simulink model "part2"  (R2025b)
settings: Solver=FixedStepAuto  StartTime=0.0  StopTime=500  FixedStep=0.1  RelTol=1e-3
values from neighbouring files (symbols this model uses):
  Aw = [zeros(3) eye(3); -diag_natwavefreq^2 -2*diag_reldampratios*diag_natwavefreq]    [NPO_init.m]    (also in kalman_init.m; passive_observer_init.m)
  Cw = [zeros(3) eye(3)]    [NPO_init.m]    (also in kalman_init.m; passive_observer_init.m)
  D = [2.6486e5 0 0 ... (first row only)    [NPO_init.m]    (also in kalman_init.m; passive_observer_init.m)
  h = 0.1    [init.m]
  K1 = [ diag([k1 k2 k3]) ... (first row only)    [NPO_init.m]    (also in passive_observer_init.m)
  K2 = diag([k7 k8 k9])    [NPO_init.m]    (also in passive_observer_init.m)
  K3 = 0.1*K4    [NPO_init.m]    (also in passive_observer_init.m = diag(diag(M) * 1e-1))
  K4 = diag([ 1000 10000 1000])    [NPO_init.m]    (also in passive_observer_init.m = diag(diag(M)))
  K_d = 2*M*Z*OMEGA_n    [init_controller.m]
  K_i = 0.1*K_p*OMEGA_n    [init_controller.m]
  K_p = M*OMEGA_n^2    [init_controller.m]
  M_inv = vesselABC.Minv([1 2 6], [1 2 6])    [NPO_init.m]    (also in kalman_init.m; passive_observer_init.m)
  T = diag([10000, 10000, 100])    [NPO_init.m]    (also in passive_observer_init.m = diag([100, 100, 100]))
  thrusters =     [thrusters_sup.mat]
  vessel =     [supply.mat]
undefined symbols (not defined in the file or in its folder): Hoerner
libraries: marine_gnc x2, marine_hydro x2
settings Model: Creator=jonbjor  LastModifiedBy=User
settings SolverCC: AlgebraicLoopSolver=TrustRegion
settings DataIOCC: ReturnWorkspaceOutputs=off
settings DebuggingCC: UnconnectedInputMsg=warning  UnconnectedOutputMsg=warning  UnconnectedLineMsg=warning  ArithmeticOperatorsInVariantConditions=warning
settings ModelReferenceCC: EnableRefExpFcnMdlSchedulingChecks=on
settings SFSimCC: SimUseLocalCustomCode=off  CustomCodeUndefinedFunction=UseInterfaceOnly
settings RTWCC: RTWUseLocalCustomCode=off  GPUComputeCapability=3.5  DLArmComputeVersion=19.05

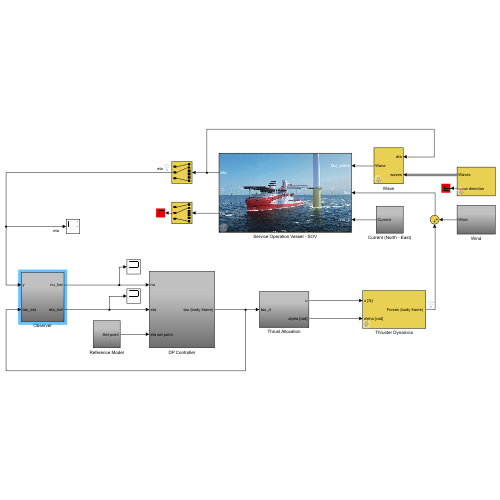
[thumbnail: Simulink's stored preview of the top-level diagram]
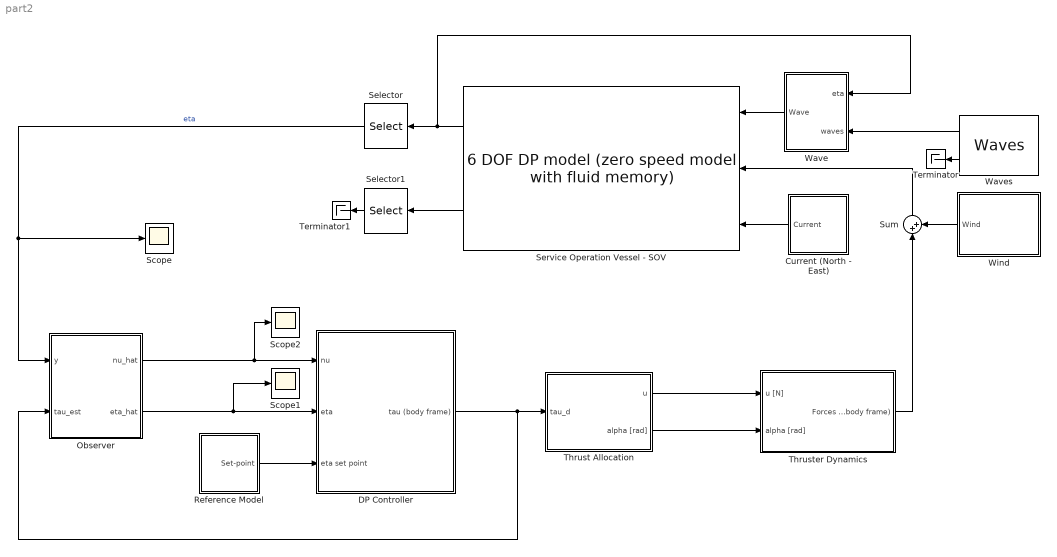
== system part2 ==
  Current (North - East) : Subsystem
  DP Controller : Subsystem
  Observer : Subsystem
  Reference Model : Subsystem
  Scope : Scope
      settings: ActiveDisplayYMinimum=-5.6386509566792773  ActiveDisplayYMaximum=19.827178567067236
  Scope1 : Scope
      settings: ActiveDisplayYMinimum=-7.2763512217109962  ActiveDisplayYMaximum=4.2414484621942279
  Scope2 : Scope
      settings: ActiveDisplayYMinimum=-5.4085848942959505  ActiveDisplayYMaximum=19.437811598484206  DataLoggingVariableName=ScopeData2
  Selector : Selector  InputPortWidth=6  IndexOptions=Index vector (dialog)  Indices=[1 2 6]  OutputSizes=1
  Selector1 : Selector  InputPortWidth=6  IndexOptions=Index vector (dialog)  Indices=[1 2 6]  OutputSizes=1
  Service Operation Vessel - SOV : marine_hydro/Hydro Library/6 DOF DP model  (zero speed model with fluid memory)  ABC=vesselABC  rho=1025  Axc=0.9*vessel.main.T*vessel.main.B  Ayc=0.9*vessel.main.T*vessel.main.Lpp  CX=1  CY_2D=Hoerner(vessel.main.B,vessel.main.T)  Bv=vessel.Bv  mask(6 DOF zero speed model){}
      link override "Integrator1 ": InitialCondition=nu0
      link override Integrator2: InitialCondition=eta0
      settings: SourceProductName=MSS Hydro
      mask Display:
      | image('SOV.jpg');
      | color('white'); port_label('output', 1, 'eta')
      | color('white'); port_label('output', 2, 'nu')
      | color('white'); port_label('input', 1, 'tau_wave')
      | color('white'); port_label('input', 2, 'tau')
      | color('white'); port_label('input', 3, 'nu_c')
  Sum : Sum  Inputs=|++
  Terminator : Terminator
  Terminator1 : Terminator
  Thrust Allocation : Subsystem
  Thruster Dynamics : Subsystem  mask{thrusterfault=off}
      mask prompts: thrusterfault "Fault on thruster #2 and #4?"
  Wave : Subsystem  mask{waveforces=on}
      mask prompts: waveforces "Waveforces enabled"
  Waves : marine_gnc/Environment/Waves/Waves  spectrum_type=ITTC  disp_flag=on  plot_spectrum=off  plot_realization=off  hs=2.5  omega_peak=2*pi/9  psi_mean=0  gamma=-1  spread=2  depth=inf  nfreq=20  ndir=10  energylim=0.005  freq_cutoff=3  dir_cutoff=0  rand_seed=123  rand_freq=on  rand_dir=on  Zeta_a=0  Omega=0  Phase=0  Wavenum=0  Psi=0
      settings: SourceProductName=MSS GNC
  Wind : Subsystem
  wires:
  Service Operation Vessel - SOV/2 -> Selector1/1
  Reference Model/1(Set-point) -> DP Controller/3(eta set point)
  DP Controller/1(tau (body frame)) -> Thrust Allocation/1(tau_d), Observer/2(tau_est)
  Service Operation Vessel - SOV/1 -> Wave/1(eta), Selector/1
  Current (North - East)/1(Current) -> Service Operation Vessel - SOV/3
  Wave/1(Wave) -> Service Operation Vessel - SOV/1
  Waves/1 -> Wave/2(waves)
  Waves/2 -> Terminator/1
  Selector1/1 -> Terminator1/1
  Observer/2(eta_hat) -> Scope1/1, DP Controller/2(eta)
  Observer/1(nu_hat) -> Scope2/1, DP Controller/1(nu)
  Thrust Allocation/1(u) -> Thruster Dynamics/1(u [N])
  Wind/1(Wind) -> Sum/2
  Thruster Dynamics/1("Forces (body frame) ") -> Sum/1
  Sum/1 -> Service Operation Vessel - SOV/2
  Thrust Allocation/2(alpha [rad]) -> Thruster Dynamics/2(alpha [rad])
  Selector/1 -> Scope/1, Observer/1(y)  "eta"

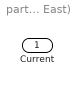
== system part2/Current (North - East) ==
  Current : Outport  VectorParamsAs1DForOutWhenUnconnected=off

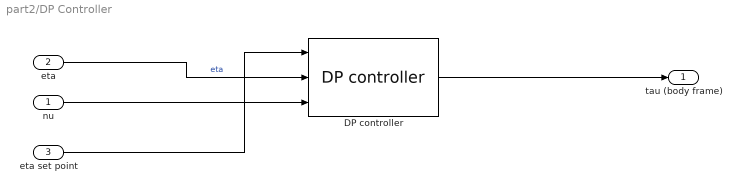
== system part2/DP Controller ==
  nu : Inport
  eta : Inport  Port=2
  eta set point : Inport  Port=3
  DP controller : marine_gnc/Control/Dynamic  Positioning /DP controller  Kp=K_p  Kd=K_d  Ki=K_i
      settings: SourceProductName=MSS GNC
  tau (body frame) : Outport  VectorParamsAs1DForOutWhenUnconnected=off
  wires:
  eta/1 -> DP controller/2  "eta"
  nu/1 -> DP controller/3
  eta set point/1 -> DP controller/1
  DP controller/1 -> tau (body frame)/1

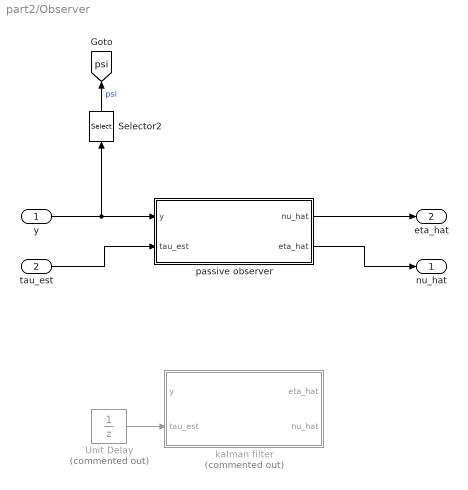
== system part2/Observer ==
  y : Inport
  tau_est : Inport  Port=2
  Selector2 : Selector  InputPortWidth=3  IndexOptions=Index vector (dialog)  Indices=[3]  OutputSizes=1
  Unit Delay : UnitDelay  Commented=on  SampleTime=h  HasFrameUpgradeWarning=on
  kalman filter : MATLAB Function  Commented=on  TreatAsAtomicUnit=on
  passive observer : Subsystem
  nu_hat : Outport  VectorParamsAs1DForOutWhenUnconnected=off
  eta_hat : Outport  Port=2  VectorParamsAs1DForOutWhenUnconnected=off
  tag scope: psi=global
  wires:
  Unit Delay/1 -> kalman filter/2(tau_est)
  Selector2/1 -> [psi]  "psi"
  y/1 -> Selector2/1, passive observer/1(y)
  passive observer/2(eta_hat) -> nu_hat/1
  passive observer/1(nu_hat) -> eta_hat/1
  tau_est/1 -> passive observer/2(tau_est)

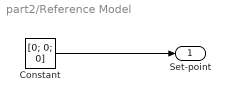
== system part2/Reference Model ==
  Constant : Constant  Value=[0; 0; 0]
  Set-point : Outport  VectorParamsAs1DForOutWhenUnconnected=off
  wires:
  Constant/1 -> Set-point/1

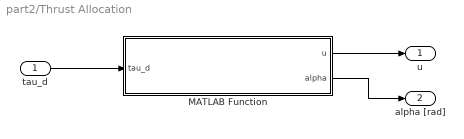
== system part2/Thrust Allocation ==
  tau_d : Inport
  MATLAB Function : MATLAB Function  TreatAsAtomicUnit=on
  u : Outport  VectorParamsAs1DForOutWhenUnconnected=off
  alpha [rad] : Outport  Port=2  VectorParamsAs1DForOutWhenUnconnected=off
  wires:
  tau_d/1 -> MATLAB Function/1(tau_d)
  MATLAB Function/1(u) -> u/1
  MATLAB Function/2(alpha) -> alpha [rad]/1

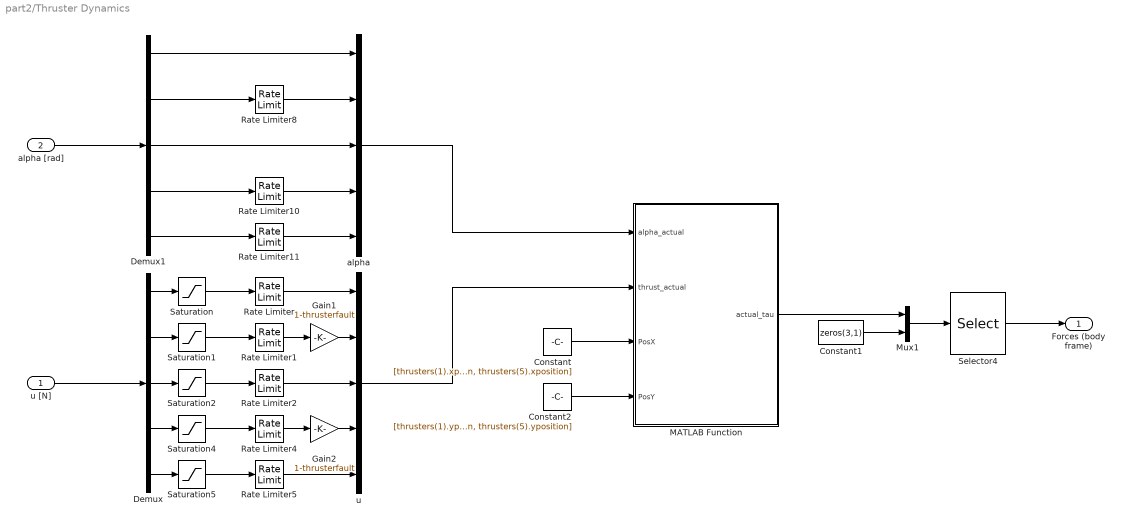
== system part2/Thruster Dynamics ==
  u [N] : Inport
  alpha [rad] : Inport  Port=2
  Constant : Constant  Value=[thrusters(1).xposition, thrusters(2).xposition, thrusters(3).xposition, thrusters(4).xposition, thrusters(5).xposition]
  Constant1 : Constant  Value=zeros(3,1)
  Constant2 : Constant  Value=[thrusters(1).yposition, thrusters(2).yposition, thrusters(3).yposition, thrusters(4).yposition, thrusters(5).yposition]
  Demux : Demux  Outputs=5
  Demux1 : Demux  Outputs=5
  Gain1 : Gain  Gain=1-thrusterfault
  Gain2 : Gain  Gain=1-thrusterfault
  MATLAB Function : MATLAB Function  TreatAsAtomicUnit=on
  Mux1 : Mux  Inputs=2
  Rate Limiter : RateLimiter  RisingSlewLimit=thrusters(1).rate  FallingSlewLimit=-thrusters(1).rate  SampleTimeMode=inherited
  Rate Limiter1 : RateLimiter  RisingSlewLimit=thrusters(2).rate  FallingSlewLimit=-thrusters(2).rate  SampleTimeMode=inherited
  Rate Limiter10 : RateLimiter  RisingSlewLimit=thrusters(4).rotationspeed  FallingSlewLimit=-thrusters(4).rotationspeed  SampleTimeMode=inherited
  Rate Limiter11 : RateLimiter  RisingSlewLimit=thrusters(5).rotationspeed  FallingSlewLimit=-thrusters(5).rotationspeed  SampleTimeMode=inherited
  Rate Limiter2 : RateLimiter  RisingSlewLimit=thrusters(3).rate  FallingSlewLimit=-thrusters(3).rate  SampleTimeMode=inherited
  Rate Limiter4 : RateLimiter  RisingSlewLimit=thrusters(4).rate  FallingSlewLimit=-thrusters(4).rate  SampleTimeMode=inherited
  Rate Limiter5 : RateLimiter  RisingSlewLimit=thrusters(5).rate  FallingSlewLimit=-thrusters(5).rate  SampleTimeMode=inherited
  Rate Limiter8 : RateLimiter  RisingSlewLimit=thrusters(2).rotationspeed  FallingSlewLimit=-thrusters(2).rotationspeed  SampleTimeMode=inherited
  Saturation : Saturate  UpperLimit=thrusters(1).thrust  LowerLimit=-thrusters(1).thrust
  Saturation1 : Saturate  UpperLimit=thrusters(2).thrust  LowerLimit=-thrusters(2).thrust
  Saturation2 : Saturate  UpperLimit=thrusters(3).thrust  LowerLimit=-thrusters(3).thrust
  Saturation4 : Saturate  UpperLimit=thrusters(4).thrust  LowerLimit=-thrusters(4).thrust
  Saturation5 : Saturate  UpperLimit=thrusters(5).thrust  LowerLimit=-thrusters(5).thrust
  Selector4 : Selector  InputPortWidth=6  IndexOptions=Index vector (dialog)  Indices=[1 2 4 5 6 3]  OutputSizes=1
  alpha : Mux  Inputs=5
  u : Mux  Inputs=5
  "Forces (body frame) " : Outport  VectorParamsAs1DForOutWhenUnconnected=off
  wires:
  Rate Limiter2/1 -> u/3
  Saturation/1 -> Rate Limiter/1
  Mux1/1 -> Selector4/1
  Constant1/1 -> Mux1/2
  Saturation4/1 -> Rate Limiter4/1
  Demux/2 -> Saturation1/1
  Saturation1/1 -> Rate Limiter1/1
  Demux/1 -> Saturation/1
  Demux/3 -> Saturation2/1
  Saturation2/1 -> Rate Limiter2/1
  Selector4/1 -> "Forces (body frame) "/1
  Gain1/1 -> u/2
  Rate Limiter1/1 -> Gain1/1
  Rate Limiter/1 -> u/1
  Rate Limiter4/1 -> Gain2/1
  Saturation5/1 -> Rate Limiter5/1
  u [N]/1 -> Demux/1
  alpha [rad]/1 -> Demux1/1
  Constant/1 -> MATLAB Function/3(PosX)
  Constant2/1 -> MATLAB Function/4(PosY)
  u/1 -> MATLAB Function/2(thrust_actual)
  alpha/1 -> MATLAB Function/1(alpha_actual)
  MATLAB Function/1(actual_tau) -> Mux1/1
  Rate Limiter10/1 -> alpha/4
  Demux1/4 -> Rate Limiter10/1
  Demux1/5 -> Rate Limiter11/1
  Rate Limiter11/1 -> alpha/5
  Demux1/1 -> alpha/1
  Gain2/1 -> u/4
  Demux/4 -> Saturation4/1
  Demux/5 -> Saturation5/1
  Rate Limiter5/1 -> u/5
  Demux1/2 -> Rate Limiter8/1
  Rate Limiter8/1 -> alpha/2
  Demux1/3 -> alpha/3

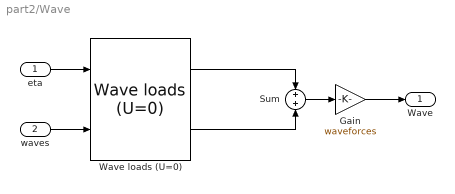
== system part2/Wave ==
  eta : Inport
  waves : Inport  Port=2
  Gain : Gain  Gain=waveforces
  Sum : Sum
  Wave loads (U=0) : marine_hydro/Hydro Library/Wave loads (U=0)  SystemSampleTime=-1  VariantActivationTime=update diagram  EmptyChoice=off  PassThrough=off  PassThroughVariantControl=(default)  EmptyChoiceVariantControl=(default)  AllowFlexibleInterface=on  Latency=0  AutoFrameSizeCalculation=off
  Wave : Outport  VectorParamsAs1DForOutWhenUnconnected=off
  wires:
  eta/1 -> Wave loads (U=0)/1
  waves/1 -> Wave loads (U=0)/2
  Sum/1 -> Gain/1
  Wave loads (U=0)/1 -> Sum/1
  Wave loads (U=0)/2 -> Sum/2
  Gain/1 -> Wave/1

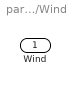
== system part2/Wind ==
  Wind : Outport  VectorParamsAs1DForOutWhenUnconnected=off

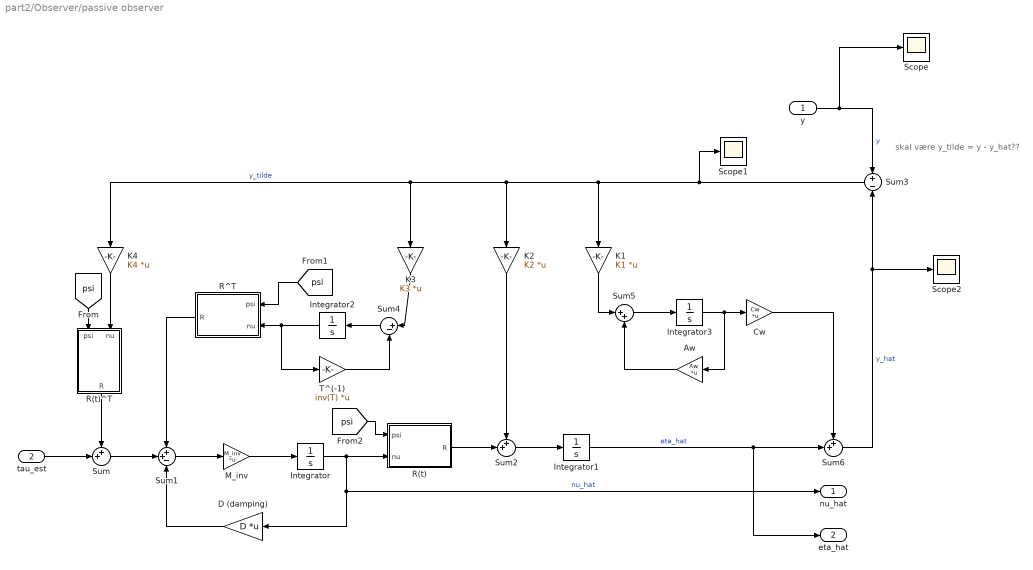
== system part2/Observer/passive observer ==
  note: skal være y_tilde = y - y_hat??
  y : Inport
  tau_est : Inport  Port=2
  Aw : Gain  Gain=Aw  Multiplication=Matrix(K*u)
  Cw : Gain  Gain=Cw  Multiplication=Matrix(K*u)
  D (damping) : Gain  Gain=D  Multiplication=Matrix(K*u)
  Integrator{,1..3} (4 alike) : Integrator
  K1 : Gain  Gain=K1  Multiplication=Matrix(K*u)
  K2 : Gain  Gain=K2  Multiplication=Matrix(K*u)
  K3 : Gain  Gain=K3  Multiplication=Matrix(K*u)
  K4 : Gain  Gain=K4  Multiplication=Matrix(K*u)
  M_inv : Gain  Gain=M_inv  Multiplication=Matrix(K*u)
  R(t) : MATLAB Function  TreatAsAtomicUnit=on
  R(t)^T : MATLAB Function  TreatAsAtomicUnit=on
  R^T : MATLAB Function  TreatAsAtomicUnit=on
  Scope : Scope
      settings: ActiveDisplayYMinimum=-5.6386509566792773  ActiveDisplayYMaximum=19.827178567067236  DataLoggingVariableName=ScopeData3
  Scope1 : Scope
      settings: ActiveDisplayYMinimum=-0.32989192595457506  ActiveDisplayYMaximum=0.716715390068409  DataLoggingVariableName=ScopeData4
  Scope2 : Scope
      settings: ActiveDisplayYMinimum=-5.4085848942959505  ActiveDisplayYMaximum=19.437811598484206  DataLoggingVariableName=ScopeData5
  Sum : Sum  Inputs=++|
  Sum1 : Sum  Inputs=++-
  Sum2 : Sum  Inputs=++|
  Sum3 : Sum  Inputs=+|-
  Sum4 : Sum  Inputs=|+-
  Sum5 : Sum  Inputs=|++
  Sum6 : Sum  Inputs=++|
  T^(-1) : Gain  Gain=inv(T)  Multiplication=Matrix(K*u)
  nu_hat : Outport  Unit=Inherit  PortDimensions=3
  eta_hat : Outport  Port=2  Unit=Inherit  PortDimensions=3
  wires:
  tau_est/1 -> Sum/2
  Sum/1 -> Sum1/2
  Sum1/1 -> M_inv/1
  M_inv/1 -> Integrator/1
  Integrator/1 -> R(t)/2(nu), D (damping)/1, nu_hat/1  "nu_hat"
  D (damping)/1 -> Sum1/3
  Sum2/1 -> Integrator1/1
  Integrator1/1 -> eta_hat/1, Sum6/2  "eta_hat"
  K2/1 -> Sum2/1
  y/1 -> Scope/1, Sum3/1  "y"
  K4/1 -> R(t)^T/2(nu)
  R(t)^T/1(R) -> Sum/1
  R(t)/1(R) -> Sum2/2
  Integrator2/1 -> T^(-1)/1, R^T/2(nu)
  Sum4/1 -> Integrator2/1
  T^(-1)/1 -> Sum4/2
  K3/1 -> Sum4/1
  R^T/1(R) -> Sum1/1
  Sum5/1 -> Integrator3/1
  Aw/1 -> Sum5/2
  K1/1 -> Sum5/1
  Integrator3/1 -> Aw/1, Cw/1
  Sum6/1 -> Scope2/1, Sum3/2  "y_hat"
  Sum3/1 -> Scope1/1, K1/1, K2/1, K3/1, K4/1  "y_tilde"
  Cw/1 -> Sum6/1
  [psi] -> R(t)^T/1(psi)
  [psi] -> R^T/1(psi)
  [psi] -> R(t)/1(psi)

== matlab function part2/Thrust Allocation/MATLAB Function ==
  data: tau_d input; u output; alpha output
function [u, alpha] = thrust_allocation_simplified(tau_d)
% INPUTS:  tau_d = [Fx; Fy; Mz] - Desired forces/moment (3x1)
% OUTPUTS: u = [u1; u2; u3; u4; u5] - Thrust magnitudes (5x1) [N]
%          alpha = [90; α2; 90; α4; α5] - Thruster angles (5x1) [deg]

%% Thruster Configuration
% Positions [m]
x = [39.3, 36.5, 34.3, -28.5, -28.5];  % x-coordinates
y = [0, 0, 0, 5, -5];                   % y-coordinates

%% Build B Matrix (3x8) - Force Decomposition
% Matrix structure: [T1, T2x, T2y, T3, T4x, T4y, T5x, T5y]
% Matrix structure: [T1, T2x, T2y, T3, T4x, T4y, T5x, T5y]
B = [
    0     1     0     0     1     0     1     0;  % Surge forces  
    1     0     1     1     0     1     0     1;  % Sway forces    
    x(1) -y(2)  x(2)  x(3) -y(4)  x(4) -y(5)  x(5)]; % Yaw moments

%% Solve using Pseudo-Inverse (Minimum-Norm Solution)
u_forces = pinv(B) * tau_d;

%% Extract Force Components
u1 = u_forces(1);      % T1 tunnel
u2x = u_forces(2);     % T2 surge component
u2y = u_forces(3);     % T2 sway component
u3 = u_forces(4);      % T3 tunnel
u4x = u_forces(5);     % T4 surge component
u4y = u_forces(6);     % T4 sway component
u5x = u_forces(7);     % T5 surge component
u5y = u_forces(8);     % T5 sway component

%% Convert to Thruster Commands
% Output vectors
u = zeros(5, 1);
alpha = zeros(5, 1);

% T1: Fixed tunnel at 90°
u(1) = u1;
alpha(1) = 90;

% T2: Variable azimuth
u(2) = sqrt(u2x^2 + u2y^2);
if u2x ~= 0 || u2y ~= 0
    alpha(2) = atan2d(u2y, u2x);
else
    alpha(2) = 0;
end

% T3: Fixed tunnel at 90°
u(3) = u3;
alpha(3) = 90;

% T4: Variable azimuth
u(4) = sqrt(u4x^2 + u4y^2);
if u4x ~= 0 || u4y ~= 0
    alpha(4) = atan2d(u4y, u4x);
else
    alpha(4) = 0;
end

% T5: Variable azimuth
u(5) = sqrt(u5x^2 + u5y^2);
if u5x ~= 0 || u5y ~= 0
    alpha(5) = atan2d(u5y, u5x);
else
    alpha(5) = 0;
end

== matlab function part2/Observer/kalman filter ==
  settings: updateMethod=DISCRETE  sampleTime=h
  data: y input; eta_hat output; tau_est input; nu_hat output
function [eta_hat, nu_hat] = kalman_filter(y, tau_est)

persistent x_prd P_prd
persistent isInitialized

if isempty(isInitialized)
    x_prd = zeros(15,1);
    P_prd = zeros(15); %eye(15)*1e-3;
    isInitialized = true;
end

h = 0.1;

M = [7.0184e6 0 0;
     0 8.5464e6 -4.4678e7;
     0 -4.5028e5 4.0505e9];
M_inv = inv(M);
D = [2.6486e5 0 0;
     0 8.8164e5 0;
     0 0 3.3774e8];

wave_period = 9*0.7;
wave_freq = 2*pi/wave_period;
diag_natwavefreq = diag([wave_freq, wave_freq, wave_freq]);
diag_reldampratios = diag([0.05, 0.05, 0.05]);

Aw = [zeros(3) eye(3); -diag_natwavefreq^2 -2*diag_reldampratios*diag_natwavefreq];
Cw = [zeros(3) eye(3)];
Ew = [zeros(3); diag([0.1, 0.1, 0.1])];

Qw   = (1e-3)*eye(3);   % wave model excitation
Qnu  = (1e-4)*eye(3);   % random walk on nu (model mismatch)
Qtau = (1e-2)*eye(3);   % unmodeled forces/moments

Q_kalman = blkdiag(Qw, Qnu, Qtau);  % 9×9
R_kalman = eye(3)*100;

eta = x_prd(7:9);
psi = eta(3);
Rpsi = [cos(psi) -sin(psi) 0;
        sin(psi)  cos(psi) 0;
        0         0        1]; 

A = [Aw zeros([6 3]) zeros([6 3]) zeros([6 3]);
     zeros([3 6]) zeros(3) zeros(3) Rpsi;
     zeros([3 6]) zeros(3) zeros(3) zeros(3);
     zeros([3 6]) zeros(3) M_inv*Rpsi.' -M_inv*D];
% M_inv*Rpsi.' skal være eye(3)???

B = [zeros([6 3]); zeros(3); zeros(3); M_inv];

C = [Cw eye(3) zeros(3) zeros(3)];

E = [Ew zeros([6 3]) zeros([6 3]);
            zeros(3) zeros(3) zeros(3);
            zeros(3) eye(3) zeros(3);
            zeros(3) zeros(3) M_inv];

Ad = eye(15) + h * A;
Bd = h * B;
Cd = C;
Ed = h * E;

Qd = Q_kalman; Rd = R_kalman;

% KF gain
K = P_prd * Cd' * inv(Cd * P_prd * Cd' + Rd);
IKC = eye(15) - K * Cd;

% Corrector: x_hat[k] and P_hat[k]
e = y - Cd * x_prd;
%e(3) = ssa(e(3));
x_hat = x_prd + K*e;
P_hat = IKC * P_prd * IKC' + K * Rd * K';

% state estimate
eta_hat = x_hat(1:3);
nu_hat = x_hat(4:6);

% Predictor: x_prd[k+1] and P_prd[k+1]
x_prd = Ad * x_hat + Bd * tau_est;
P_prd = Ad * P_hat * Ad' + Ed * Qd * Ed';

== matlab function part2/Observer/passive observer/R(t)^T ==
  data: psi input; nu input; R output
function R = fcn(psi,nu)

Rpsi = [cos(psi) -sin(psi) 0;
        sin(psi)  cos(psi) 0;
        0         0        1];

R = transpose(Rpsi) * nu;

== matlab function part2/Thruster Dynamics/MATLAB Function ==
  data: alpha_actual input; thrust_actual input; actual_tau output; PosX input; PosY input
function actual_tau   = fcn(alpha_actual,thrust_actual,PosX,PosY)

    Alpha_surge =[cos(alpha_actual(1)) cos(alpha_actual(2)) cos(alpha_actual(3)) cos(alpha_actual(4)) cos(alpha_actual(5))];  
    Alpha_sway = [sin(alpha_actual(1)) sin(alpha_actual(2)) sin(alpha_actual(3)) sin(alpha_actual(4)) sin(alpha_actual(5))];
    Alpha_yaw = [sin(alpha_actual(1))*PosX(1)-cos(alpha_actual(1))*PosY(1) sin(alpha_actual(2))*PosX(2)-cos(alpha_actual(2))*PosY(2) ...
                 sin(alpha_actual(3))*PosX(3)-cos(alpha_actual(3))*PosY(3) sin(alpha_actual(4))*PosX(4)-cos(alpha_actual(4))*PosY(4) ...
                 sin(alpha_actual(5))*PosX(5)-cos(alpha_actual(5))*PosY(5)];

    actual_tau = [Alpha_surge; Alpha_sway; Alpha_yaw]*thrust_actual;
end

== matlab function part2/Observer/passive observer/R^T ==
  data: psi input; nu input; R output
function R = fcn(psi,nu)

Rpsi = [cos(psi) -sin(psi) 0;
        sin(psi)  cos(psi) 0;
        0         0        1];

R = transpose(Rpsi) * nu;

== matlab function part2/Observer/passive observer/R(t) ==
  data: psi input; nu input; R output
function R = fcn(psi,nu)

Rpsi = [cos(psi) -sin(psi) 0;
        sin(psi)  cos(psi) 0;
        0         0        1];

R = Rpsi * nu;
